simulink model "single_panel_mppt_sim"  (R2021b)
settings: Solver=ode23tb  StartTime=0.0  StopTime=sim_time  FixedStep=5e-5  MaxStep=max_time_step  RelTol=1e-3
values from neighbouring files (symbols this model uses):
  actions = (-1:1) * duty_step    [deep_q_mppt_test.m]    (also in single_panel_mppt.m)
  alpha = 0.1    [single_panel_mppt.m]
  deg_threshold = deg2rad(5)    [single_panel_mppt.m]
  exploration_factor_init = 0.9999    [single_panel_mppt.m]
  gamma = 0.9    [deep_q_mppt_test.m]    (also in single_panel_mppt.m)
  Isc = 5.17    [deep_q_mppt_test.m]    (also in single_panel_mppt.m)
  n_I = 100    [single_panel_mppt.m]
  n_V = 100    [single_panel_mppt.m]
  Ts = 1e-4    (= 0.0001)    [deep_q_mppt_test.m]    (also in signle_panel_mppt.m = 0.001; single_panel_mppt.m)
  Voc = 43.99    [deep_q_mppt_test.m]    (also in signle_panel_mppt.m; single_panel_mppt.m)
  wn = 4    [deep_q_mppt_test.m]    (also in single_panel_mppt.m)
  wp = 1    [deep_q_mppt_test.m]    (also in single_panel_mppt.m)
undefined symbols (not defined in the file or in its folder): irr_data, mpp_data
libraries: spsControlledVoltageSourceLib x1, spsDiodeLib x1, simulink x1, spsPVArrayLib x1, spspowerguiLib x1
settings Model: Creator=HP  LastModifiedBy=HP

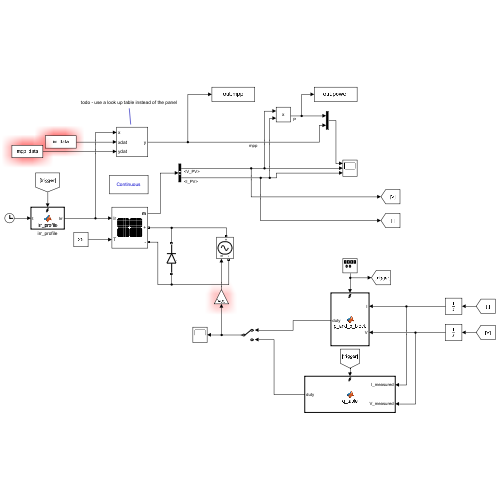
[thumbnail: Simulink's stored preview of the top-level diagram]
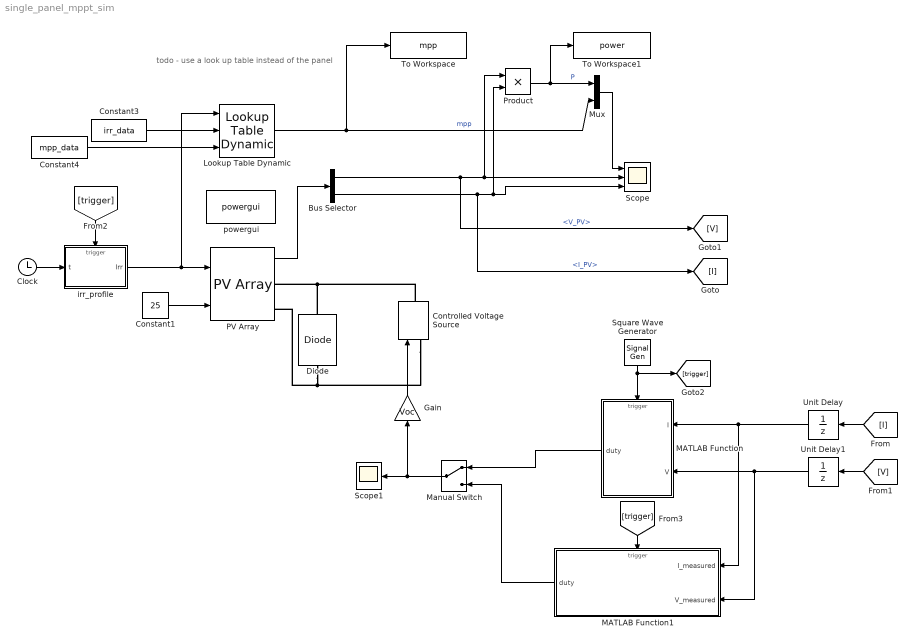
== system single_panel_mppt_sim ==
  note: todo - use a look up table instead of the panel
  Bus Selector : BusSelector  OutputSignals=V_PV,I_PV
  Clock : Clock
  Constant1 : Constant  Value=25
  Constant3 : Constant  Value=irr_data
  Constant4 : Constant  Value=mpp_data
  Controlled Voltage Source : spsControlledVoltageSourceLib/Controlled Voltage Source  Initialize=on  Source_Type=DC  Amplitude=0  Phase=0  Frequency=0  Measurements=None
  Diode : spsDiodeLib/Diode  Ron=0  Lon=0  Vf=0.8  IC=0  UseSnubber=0  Rs=0  Cs=0  Measurements=off
  Gain : Gain  Gain=Voc
  Lookup Table Dynamic : simulink/Lookup Tables/Lookup Table Dynamic  LookUpMeth=Interpolation-Use End Values  OutDataType=fixdt('double')  OutScaling=[]  OutputDataTypeScalingMode=Specify via dialog  OutDataTypeStr=double  DoSatur=off
  MATLAB Function : MATLAB Function  TreatAsAtomicUnit=on
  MATLAB Function1 : MATLAB Function  TreatAsAtomicUnit=on
  Manual Switch : ManualSwitch
  Mux : Mux  Inputs=2
  PV Array : spsPVArrayLib/PV Array  Npar=1  Nser=1  PlotType=array @ 1000 W/m2 & specified temperatures  S_vec="[ 1000  500  100 ]"  Temp_C_vec="[ 45 25  ]"  ModuleName=A10Green Technology A10J-S72-175  PlotWhenSelected=off  Pm=175.0914  Ncell=72  Voc=43.99  Isc=5.17  Vm=36.63  Im=4.78  beta_Voc_pc=-0.3616  alpha_Isc_pc=0.041509  beta_Voc=-0.15907  alpha_Isc=0.002146  IL=5.178  I0=1.7842e-10  nI=0.98852  Rsh=249.6758  Rs=0.38412  RobustModel=off  RobustCellTemperature=313.3991  BAL=off  Tc=1e-6  Tfilter=1e-5
  Product : Product
  Scope : Scope  NumInputPorts=3
  Scope1 : Scope
  Square Wave Generator : SignalGenerator  WaveForm=square  Frequency=1/Ts
  To Workspace : ToWorkspace  VariableName=mpp  SaveFormat=Timeseries  SampleTime=-1
  To Workspace1 : ToWorkspace  VariableName=power  SaveFormat=Timeseries  SampleTime=-1
  Unit Delay : UnitDelay  SampleTime=-1  HasFrameUpgradeWarning=on
  Unit Delay1 : UnitDelay  SampleTime=-1  HasFrameUpgradeWarning=on
  irr_profile : MATLAB Function  TreatAsAtomicUnit=on
  powergui : spspowerguiLib/powergui  Priority=1  SimulationMode=Continuous  SampleTime=50e-6  frequency=60  Iterations=50  frequencyindice=0  Pbase=100e6  ErrMax=1e-4  UnitsV=kV  UnitsW=MW  buscounter=0  FunctionMessages=off  echomessages=off  EnableUseOfTLC=off  CurrentSourceSwitches=off  DisableSnubberDevices=off  DisableRonSwitches=off  DisableVfSwitches=off  DisplayEquations=off  AutomaticDiscreteSolvers=off  SolverType=Tustin/Backward Euler (TBE)  Interpol=off  ExternalGateDelay=off  methode=off  Ts=100  x0status=blocks  SPID=on  SwTol=0  HookPort=off  NonlinearTolerance=1e-4  nMaxIteration=100  ContinueOnMaxIteration=off  RestoreLinks=warning  ResistiveCurrentMeasurement=off  Frange=[0:2:500]  Ylog=off  Xlog=on  ShowGrid=off  save=off  variable=ZData  structure=0  ZoomFFT=off  StartTime=0.0  cycles=1  DisplayStyle=1  fundamental=60  FreqAxis=off  MaxFrequency=1000  frequencyindicesteady=1  RmsSteady=1  display=off
  wires:
  Constant1/1 -> PV Array/2
  PV Array/1 -> Bus Selector/1
  Bus Selector/1 -> [V], Product/1, Scope/2  "<V_PV>"
  Bus Selector/2 -> [I], Scope/3, Product/2  "<I_PV>"
  [I] -> Unit Delay/1
  [V] -> Unit Delay1/1
  Gain/1 -> Controlled Voltage Source/1
  Product/1 -> To Workspace1/1, Mux/1  "P"
  Mux/1 -> Scope/1
  irr_profile/1(Irr) -> Lookup Table Dynamic/1, PV Array/1
  Lookup Table Dynamic/1 -> To Workspace/1, Mux/2  "mpp"
  Constant3/1 -> Lookup Table Dynamic/2
  Constant4/1 -> Lookup Table Dynamic/3
  Clock/1 -> irr_profile/1(t)
  Square Wave Generator/1 -> MATLAB Function/Trigger, [trigger]
  [trigger] -> irr_profile/Trigger
  [trigger] -> MATLAB Function1/Trigger
  Unit Delay1/1 -> MATLAB Function1/2(V_measured), MATLAB Function/2(V)
  Unit Delay/1 -> MATLAB Function1/1(I_measured), MATLAB Function/1(I)
  MATLAB Function/1(duty) -> Manual Switch/1
  MATLAB Function1/1(duty) -> Manual Switch/2
  Manual Switch/1 -> Scope1/1, Gain/1
  connections:
  Diode/LConn1 -- Controlled Voltage Source/LConn1 -- PV Array/RConn2
  Diode/RConn1 -- Controlled Voltage Source/RConn1 -- PV Array/RConn1

== matlab function single_panel_mppt_sim/irr_profile ==
  data: t input; Irr output
  events: trigger input RISING_EDGE_EVENT
function Irr = irr_profile(t)
%#codegen

%    This function was generated by the Symbolic Math Toolbox version 9.0.
%    12-Jan-2022 21:25:19

t2 = ((0.0 <= t) & (t <= 2.0./5.0));
t3 = ((2.0./5.0 <= t) & (t <= 4.0./5.0));
t4 = ((4.0./5.0 <= t) & (t <= 6.0./5.0));
t5 = ((6.0./5.0 <= t) & (t <= 7.0./5.0));
t6 = ((7.0./5.0 <= t) & (t <= 9.0./5.0));
t7 = ((t <= 2.0) & (9.0./5.0 <= t));
t8 = t.*1.25e+3-1.0e+2;
if (t2)
    Irr = 5.0e+2;
elseif (t3)
    Irr = t8;
elseif (t4)
    Irr = 8.0e+2;
elseif (t5)
    Irr = t8.*-2.0+3.6e+3;
elseif (t6)
    Irr = t.*5.0e+2+t8-2.05e+3;
elseif (t7)
    Irr = 1.0e+3;
else
    Irr = NaN;
end

== matlab function single_panel_mppt_sim/MATLAB Function ==
  data: I input; duty output; V input; duty_step parameter
  events: trigger input RISING_EDGE_EVENT
% @p_and_o - a function implementing the Perturb and Observe MPPT algorithm
function duty = p_and_o_block(I, V, duty_step)

    % make sure that function is included in the project path
    duty = 0; % a requried init so that the program knows the size of the var
    duty = p_and_o(I, V, duty_step);    
end

== matlab function single_panel_mppt_sim/MATLAB Function1 ==
  data: I_measured input; duty output; V_measured input; Voc parameter; Isc parameter; deg_threshold parameter; wp parameter; wn parameter; n_V parameter; n_I parameter; actions parameter; alpha parameter; gamma parameter; exploration_factor_init parameter
  events: trigger input RISING_EDGE_EVENT
function duty = q_table(I_measured, V_measured, Voc, Isc, deg_threshold, wp, wn, n_V, n_I, actions, alpha, gamma, exploration_factor_init)
    
    % normalize
    I = I_measured / Isc;
    V = V_measured / Voc;
    
    % init
    persistent I_old V_old deg_old duty_old Q_table action_old exploration_factor
    if isempty(I_old)
        I_old = 0;
        V_old = 0;
        deg_old = 2;
        duty_old = 0;
        exploration_factor = exploration_factor_init;

        Q_table = zeros(n_V, n_I, 2, length(actions));
        
        % pick the middle action as an initialization
        if mod(length(actions), 2) == 0
            action_old = length(actions) / 2;
        else
            action_old = (length(actions) + 1) / 2;
        end
    end
    
    % calc changes
    dI = I - I_old;
    dV = V - V_old;
    dP = V * I - V_old * I_old;
    
    % see where deg is (are we close to the MPP or not?)
    deg = atan(dI / dV) + atan(I / V);
    
    if abs(deg) > deg_threshold
        deg = 2;    % far form the MPP
    else
        deg = 1;    % close to the MPP
    end
    
    % calc reward
    if dP > 0
        R = wp * dP;
    else
        R = wn * dP;
    end
    
    V_index = round(interp1([0,1], [1, n_V], V));
    V_old_index = round(interp1([0,1], [1, n_V], V_old));

    I_index = round(interp1([0,1], [1, n_I], I));
    I_old_index = round(interp1([0,1], [1, n_I], I_old));
    
    % update Q
    Q_table(V_old_index, I_old_index, deg_old, action_old) = (1 - alpha) * ... 
    Q_table(V_old_index, I_old_index, deg_old, action_old) + ...
        alpha * (R + gamma * max(Q_table(V_index, I_index, deg, :)));

    
    % exploration VS exploitation
    if rand < exploration_factor
        action_old = randi(length(actions));
    else
        [~, argmax] = max(Q_table(V_index, I_index, deg, :));
        action_old = argmax;
    end

    duty = duty_old + actions(action_old);

    if duty > 1 || duty < 0
        duty = duty_old;
    end

    % update old values
    V_old = V;
    I_old = I;
    deg_old = deg;
    duty_old = duty;
    exploration_factor = exploration_factor * exploration_factor_init;
end
